simulink model "ChCs_of_Sensor_Accelerator_Pedal"  (R2021a)
settings: Solver=FixedStepAuto  StartTime=0.0  StopTime=10  RelTol=1e-3
settings Model: Creator=lenovo  LastModifiedBy=lenovo
settings DataIOCC: LoadExternalInput=on

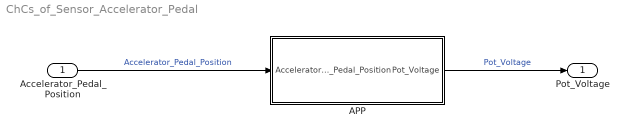
== system ChCs_of_Sensor_Accelerator_Pedal ==
  Accelerator_Pedal_Position : Inport
  APP : Subsystem
  Pot_Voltage : Outport
  wires:
  APP/1(Pot_Voltage) -> Pot_Voltage/1  "Pot_Voltage"
  Accelerator_Pedal_Position/1 -> APP/1(Accelerator_Pedal_Position)  "Accelerator_Pedal_Position"

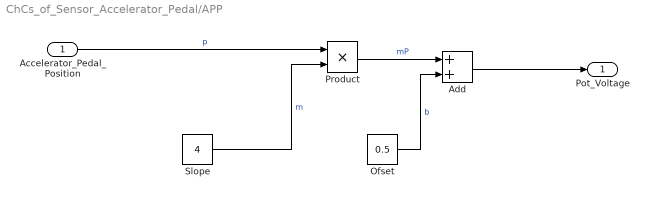
== system ChCs_of_Sensor_Accelerator_Pedal/APP ==
  Accelerator_Pedal_Position : Inport
  Add : Sum
  Ofset : Constant  Value=0.5
  Product : Product
  Slope : Constant  Value=4
  Pot_Voltage : Outport
  wires:
  Add/1 -> Pot_Voltage/1
  Product/1 -> Add/1  "mP"
  Slope/1 -> Product/2  "m"
  Ofset/1 -> Add/2  "b"
  Accelerator_Pedal_Position/1 -> Product/1  "p"
